simulink model "darko_model"  (R2020b)
settings: Solver=VariableStepAuto  StartTime=0.0  StopTime=1.8  RelTol=1e-3
values from neighbouring files (symbols this model uses):
  x_eq = [[0; 0; 0]; [0; 0; 0]; [1/sqrt(2); 0; -1/sqrt(2);0]; [0; 0; 0]]    [main_linearisation_rot.m]
settings Model: Creator=florian  LastModifiedBy=florian

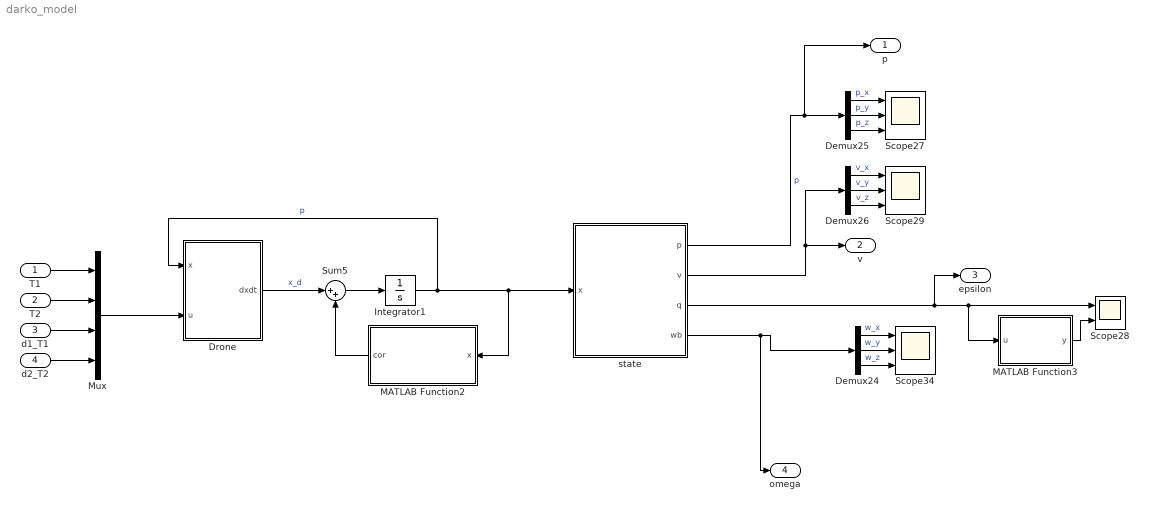
== system darko_model ==
  T1 : Inport
  T2 : Inport  Port=2
  d1_T1 : Inport  Port=3
  d2_T2 : Inport  Port=4
  Demux24 : Demux  Outputs=3
  Demux25 : Demux  Outputs=3
  Demux26 : Demux  Outputs=3
  Drone : MATLAB Function  TreatAsAtomicUnit=on
  Integrator1 : Integrator  InitialCondition=x_eq
  MATLAB Function2 : MATLAB Function  TreatAsAtomicUnit=on
  MATLAB Function3 : MATLAB Function  TreatAsAtomicUnit=on
  Mux : Mux
  Scope27 : Scope  NumInputPorts=3
  Scope28 : Scope  NumInputPorts=2
  Scope29 : Scope  NumInputPorts=3
  Scope34 : Scope  NumInputPorts=3
  Sum5 : Sum  Inputs=|++
  state : MATLAB Function  TreatAsAtomicUnit=on
  p : Outport  VectorParamsAs1DForOutWhenUnconnected=off
  v : Outport  Port=2  VectorParamsAs1DForOutWhenUnconnected=off
  epsilon : Outport  Port=3  VectorParamsAs1DForOutWhenUnconnected=off
  omega : Outport  Port=4  VectorParamsAs1DForOutWhenUnconnected=off
  wires:
  Sum5/1 -> Integrator1/1
  MATLAB Function2/1(cor) -> Sum5/2
  Drone/1(dxdt) -> Sum5/1  "x_d"
  Integrator1/1 -> Drone/1(x), state/1(x), MATLAB Function2/1(x)  "p"
  Demux25/3 -> Scope27/3  "p_z"
  Demux26/2 -> Scope29/2  "v_y"
  Demux24/1 -> Scope34/1  "w_x"
  MATLAB Function3/1(y) -> Scope28/2
  state/3(q) -> epsilon/1, MATLAB Function3/1(u), Scope28/1
  Demux25/1 -> Scope27/1  "p_x"
  state/4(wb) -> omega/1, Demux24/1
  Demux24/2 -> Scope34/2  "w_y"
  state/1(p) -> p/1, Demux25/1  "p"
  Demux24/3 -> Scope34/3  "w_z"
  state/2(v) -> v/1, Demux26/1
  Demux25/2 -> Scope27/2  "p_y"
  Demux26/3 -> Scope29/3  "v_z"
  Demux26/1 -> Scope29/1  "v_x"
  Mux/1 -> Drone/2(u)
  T2/1 -> Mux/2
  T1/1 -> Mux/1
  d1_T1/1 -> Mux/3
  d2_T2/1 -> Mux/4

== matlab function darko_model/Drone ==
  data: x input; u input; dxdt output; drone parameter
function dxdt  = drone(x, u, drone)

%% physical constants
% gravity
g = drone.G;
% vehicle mass
m = drone.MASS;
% vehicle inertia matrix
J = drone.INERTIA; % [3x3 real symmetric] in body axis

%% state demultiplexing
% p = x(1:3);
v = x(4:6);
q  = x(7:10);
wb = x(11:13);

Rq = q2dcm(q);
wind = 0;
[Fp, Mp] = external_force_moment(x, u, wind, drone);

% position
dpdt = v;

% kinematics
dvdt =  -[0;0;g] + (1/m)*Rq*drone.Fb*u;% + (1/m)*Rq*Fp; 

%% quaternion derivative
eta = q(1);
eps = q(2:4);

dqdt = (1/2)*[-eps'; eta*eye(3) + skew_sym(eps)]*wb;

%% angular velocity derivative
% kinematics
dwdt = -J\cross(wb, J*wb) + J\(drone.Mb*u);% + J\Mp;


%% derivative multiplexing
dxdt = [dpdt; dvdt; dqdt; dwdt] ;

== matlab function darko_model/MATLAB Function2 ==
  data: x input; cor output
function cor  = fcn(x)
%#codegen
q  = x(7:10);
n = norm(q);
mismatch = 1-n;
cor = [0;0;0; 0;0;0; mismatch*q; 0;0;0];

== matlab function darko_model/MATLAB Function3 ==
  data: u input; y output
function y = fcn(u)
%#codegen

y = norm(u);

== matlab function darko_model/state ==
  data: x input; p output; v output; q output; wb output
function [p, v, q, wb] = demux(x)
%#codegen

p = x(1:3);
v = x(4:6);
q  = x(8:10);
wb = x(11:13);
